simulink model "przestrzen_stanu_dys"  (R2014b)
settings: Solver=ode45  StartTime=0.0  StopTime=Tsym  RelTol=1e-3
undefined symbols (not defined in the file): A, alfa, Az, Bz, Cz, deltaFc, deltaFd, deltaFh, deltaTc, deltaTd, deltaTh, Dz, Fc, Fd, Fh, Fh0, h0, T0, tau, tauh, Tc, Td, Th, Tp, Tskok
settings Model: Creator=Arek  LastModifiedBy=Arek
settings DebuggingCC: SolverPrmCheckMsg=none

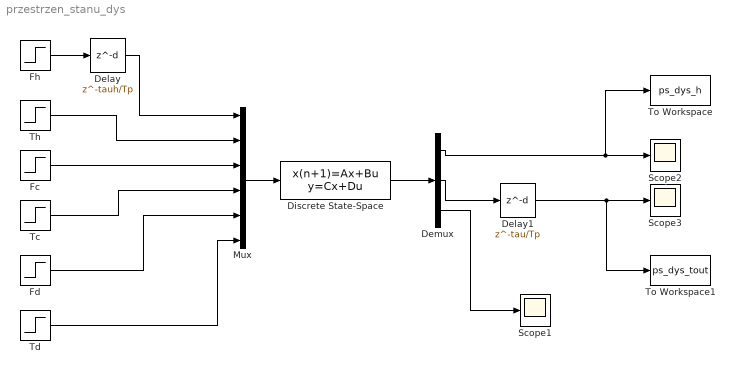
== system przestrzen_stanu_dys ==
  Delay : Delay  DelayLength=tauh/Tp  InitialCondition=Fh0  SampleTime=Tp
  Delay1 : Delay  DelayLength=tau/Tp  InitialCondition=T0  SampleTime=Tp
  Demux : Demux  Outputs=3
  Discrete State-Space : DiscreteStateSpace  A=Az  B=Bz  C=Cz  D=Dz  X0=[h0,T0,-alfa*sqrt(h0)/(2*A)]  SampleTime=Tp
  Fc : Step  Time=Tskok  Before=Fc  After=Fc+deltaFc  SampleTime=Tp
  Fd : Step  Time=Tskok  Before=Fd  After=Fd+deltaFd  SampleTime=Tp
  Fh : Step  Time=Tskok  Before=Fh  After=Fh+deltaFh  SampleTime=Tp
  Mux : Mux  Inputs=6
  Scope1 : Scope
  Scope2 : Scope
      settings: SaveName=ScopeData2
  Scope3 : Scope
      settings: SaveName=ScopeData3
  Tc : Step  Time=Tskok  Before=Tc  After=Tc+deltaTc  SampleTime=Tp
  Td : Step  Time=Tskok  Before=Td  After=Td+deltaTd  SampleTime=Tp
  Th : Step  Time=Tskok  Before=Th  After=Th+deltaTh  SampleTime=Tp
  To Workspace : ToWorkspace  VariableName=ps_dys_h  SaveFormat=Timeseries  SampleTime=-1
  To Workspace1 : ToWorkspace  VariableName=ps_dys_tout  SaveFormat=Timeseries  SampleTime=-1
  wires:
  Mux/1 -> Discrete State-Space/1
  Discrete State-Space/1 -> Demux/1
  Demux/1 -> To Workspace/1, Scope2/1
  Delay1/1 -> To Workspace1/1, Scope3/1
  Demux/2 -> Delay1/1
  Fh/1 -> Delay/1
  Delay/1 -> Mux/1
  Th/1 -> Mux/2
  Fc/1 -> Mux/3
  Tc/1 -> Mux/4
  Fd/1 -> Mux/5
  Td/1 -> Mux/6
  Demux/3 -> Scope1/1
